simulink model "ec_single_vs_fixed"  (Simulink 10.0)
settings: Solver=FixedStepDiscrete  StartTime=0.0  StopTime=10  RelTol=1e-3
InitFcn:
  | ec_single_vs_fixed_data;
StartFcn:
  | tic;
StopFcn:
  | toc;
undefined symbols (not defined in the file): dfilt, ec_length, Fs, pic_frame_size, sm_length, spkr_to_mic_delay
libraries: dspsrcs4 x6, dspsigops x5, simulink x4, dspsnks4 x3, dspadpt3 x2, dsparch4 x1
settings Model: Creator=Kerry Schutz  LastModifiedBy=bhisma
settings DataIOCC: LimitDataPoints=on  SignalLoggingSaveFormat=ModelDataLogs
settings OptimizationCC: BlockReduction=off  DefaultParameterBehavior=Inlined  InlineInvariantSignals=on  ExpressionDepthLimit=2147483647  StateBitsets=on  DataBitsets=on  ZeroExternalMemoryAtStartup=off  ZeroInternalMemoryAtStartup=off  EfficientFloat2IntCast=on  LifeSpan=1  EfficientTunableParamExpr=on
settings DebuggingCC: AlgebraicLoopMsg=none  SaveWithParameterizedLinksMsg=none  SolverPrmCheckMsg=warning  ParameterPrecisionLossMsg=none  FcnCallInpInsideContextMsg=warning  StateNameClashWarn=warning
settings HardwareCC: ProdBitPerInt=16  ProdBitPerPointer=16  ProdBitPerSizeT=16  ProdBitPerPtrDiffT=16  ProdIntDivRoundTo=Zero  ProdEndianess=LittleEndian  ProdWordSize=16  ProdHWDeviceType=Microchip->dsPIC  TargetHWDeviceType=32-bit Generic
settings SFSimCC: SimUseLocalCustomCode=on  SimParseCustomCode=off  MATLABDynamicMemAlloc=off  CustomCodeUndefinedFunction=FilterOut
settings RTWCC: Description=Real-Time Workshop Embedded Coder (no auto configuration)  SystemTargetFile=ert.tlc  GenCodeOnly=on  TemplateMakefile=ert_default_tmf  RTWUseLocalCustomCode=on  CreateSILPILBlock=SIL
settings CodeAppCC: IgnoreCustomStorageClasses=off  CustomSymbolStrType=$N$R$M  InternalIdentifier=Classic  InlinedPrmAccess=Macros
settings ERTTargetCC: TargetFcnLib=ansi_tfl_tmw.mat  GenerateSampleERTMain=on  IncludeMdlTerminateFcn=off  SupportAbsoluteTime=off  PurelyIntegerCode=on  SupportNonFinite=off  SupportComplex=off  InlinedParameterPlacement=NonHierarchical  ERTCustomFileTemplate=example_file_process.tlc  ConvertIfToSwitch=off  SuppressUnreachableDefaultCases=off

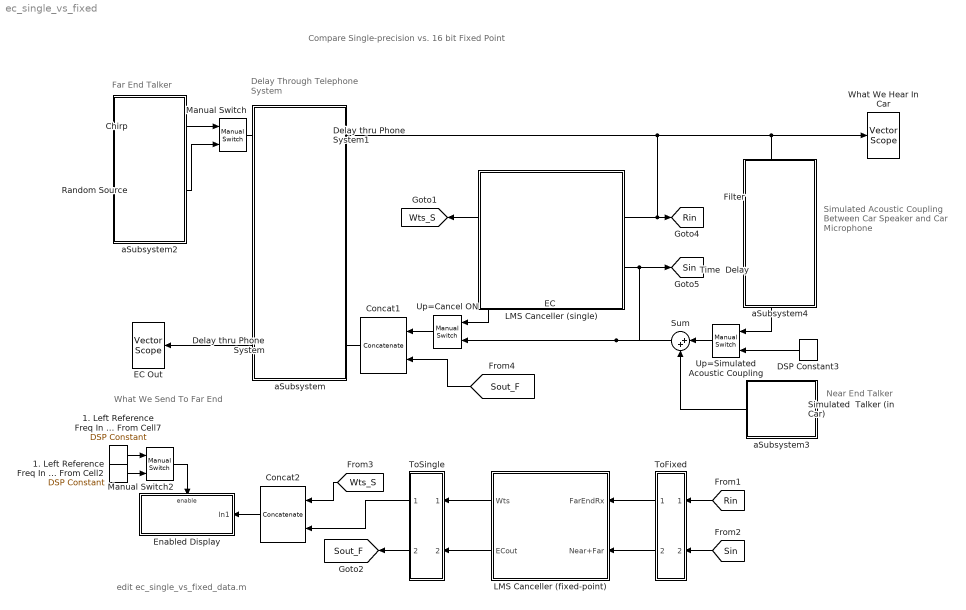
== system ec_single_vs_fixed ==
  note: Compare Single-precision vs. 16 bit Fixed Point
  note: Delay Through
      | Telephone System
  note: Simulated Acoustic
      | Coupling
      | Between Car Speaker
      | and
      | Car Microphone
  note: Far End Talker
  note: Near
      | End
      | Talker
  note: What We Send To
      | Far End
  note: edit ec_single_vs_fixed_data.m
  1. Left Reference Freq In Hz From Cell2 : dspsrcs4/DSP Constant  SystemSampleTime=-1  Value=0  SampleMode=Discrete  discreteOutput=Sample-based  continuousOutput=Sample-based  sampTime=pic_frame_size/Fs  framePeriod=pic_frame_size/Fs  dataType=int16  isSigned=on  wordLen=16  udDataType=sfix(16)  fracBitsMode=Best precision  numFracBits=15  InterpretAs1D=-inf  Ts=-inf  FramebasedOutput=-inf
      settings: SourceProductName=DSP System Toolbox  SourceProductBaseCode=DS  additionalParams=on
  1. Left Reference Freq In Hz From Cell7 : dspsrcs4/DSP Constant  SystemSampleTime=-1  Value=1  SampleMode=Discrete  discreteOutput=Sample-based  continuousOutput=Sample-based  sampTime=pic_frame_size/Fs  framePeriod=pic_frame_size/Fs  dataType=int16  isSigned=on  wordLen=16  udDataType=sfix(16)  fracBitsMode=Best precision  numFracBits=15  InterpretAs1D=-inf  Ts=-inf  FramebasedOutput=-inf
      settings: SourceProductName=DSP System Toolbox  SourceProductBaseCode=DS  additionalParams=on
  Chirp : dspsrcs4/Chirp  sweep=Linear  mode=Unidirectional  f0=100  f1=4000  t1=pic_frame_size/Fs  Tsweep=pic_frame_size/Fs  phase=0  Ts=1/Fs  spf=pic_frame_size  datatype=Single
      settings: SourceProductName=DSP System Toolbox
  Concat1 : Concatenate  Mode=Multidimensional array  ConcatenateDimension=2
  Concat2 : Concatenate  Mode=Multidimensional array  ConcatenateDimension=2
  DSP Constant3 : dspsrcs4/DSP Constant  SystemSampleTime=-1  Value=0  SampleMode=Discrete  discreteOutput=Sample-based  continuousOutput=Sample-based  sampTime=pic_frame_size/Fs  framePeriod=pic_frame_size/Fs  dataType=single  isSigned=on  wordLen=16  udDataType=sfix(16)  fracBitsMode=Best precision  numFracBits=15  InterpretAs1D=off  Ts=pic_frame_size/Fs  FramebasedOutput=off
      settings: SourceProductName=DSP System Toolbox  SourceProductBaseCode=DS
  Delay thru Phone System : dspsigops/Delay  dly_unit=Samples  delay=100  ic_detail=off  dif_ic_for_ch=off  dif_ic_for_dly=off  ic=0  reset_popup=None
      settings: SourceProductName=DSP System Toolbox  SourceProductBaseCode=DS
  Delay thru Phone System1 : dspsigops/Delay  dly_unit=Samples  delay=100  ic_detail=off  dif_ic_for_ch=off  dif_ic_for_dly=off  ic=0  reset_popup=None
      settings: SourceProductName=DSP System Toolbox  SourceProductBaseCode=DS
  EC : Subsystem
  EC Out : dspsnks4/Vector Scope  ScopeProperties=on  Domain=Time  HorizSpan=4  DisplayProperties=off  AxisGrid=on  Memory=off  FrameNumber=on  AxisLegend=on  AxisZoom=off  OpenScopeAtSimStart=on  OpenScopeImmediately=off  FigPos=[285 420 306 206]  AxisProperties=off  XUnits=Hertz  XRange=[0...Fs/2]  InheritXIncr=on  XIncr=1  XLabel=Time  XLimit=Auto  XMin=0  XMax=1  XStart=0  YUnits=dB  YLabel=Amplitude  LineProperties=off  LineColors=[1 0 0]|[0 1 0]
      settings: SourceProductName=DSP System Toolbox  SourceProductBaseCode=DS  YMin=-0.526783668994904  YMax=0.550434925854206
  Enabled Display : Subsystem  TreatAsAtomicUnit=on
  Filter : dsparch4/Digital Filter  Tag=BlockMethodSubSystem  TypePopup=FIR (all zeros)  IIRFiltStruct=Direct form II transposed  AllPoleFiltStruct=Direct form  FIRFiltStruct=Direct form  CoeffSource=Specify via dialog  NumCoeffs=spkr_to_mic_filter  DenCoeffs=[1 0.1]  BiQuadCoeffs=[1 0.3 0.4 1 0.1 0.2]  LatticeCoeffs=[0.2 0.4]  denIgnore=on  FiltPerSampPopup=One filter per frame  IC=0  ICnum=0  ICden=0  roundingMode=Floor  overflowMode=off  ScaleValues=1  scaleValueFracLength=14  stageInFracLength=15  stageOutFracLength=15  FilterSource=Specify via dialog  dfiltObjectName=dfilt.dffir([1 2 1])
      settings: SourceProductName=DSP System Toolbox  SourceProductBaseCode=DS
  LMS Canceller (fixed-point) : Subsystem  DataTypeOverride=Double  MinMaxOverflowLogging=MinMaxAndOverflow
  LMS Canceller (single) : Subsystem
      mask Display: disp('')
  Manual Switch : simulink/Signal Routing/Manual Switch  SystemSampleTime=-1  sw=0  action=0  varsize=off
      settings: SourceProductName=Simulink  SourceProductBaseCode=SL
  Manual Switch2 : simulink/Signal Routing/Manual Switch  SystemSampleTime=-1  sw=1  action=0  varsize=off
      settings: SourceProductName=Simulink  SourceProductBaseCode=SL
  Random Source : dspsrcs4/Random Source  SrcType=Gaussian  NormMethod=Ziggurat  CltLength=12  MinVal=0  MaxVal=1  MeanVal=0  VarVal=.2  RepMode=Repeatable  rawSeed=1  IsInherit=off  SampMode=Discrete  SampTime=1/Fs  SampFrame=pic_frame_size  DataType=Single  OutComplex=Real
  Simulated  Talker (in Car) : dspsrcs4/Sine Wave  Amplitude=0.2  Frequency=102  Phase=0  SampleMode=Discrete  OutComplex=Real  CompMethod=Trigonometric fcn  TableSize=Speed  SampleTime=1/Fs  SamplesPerFrame=pic_frame_size  dataType=single  wordLen=16  udDataType=sfix(16)  fracBitsMode=Best precision  numFracBits=15  ResetState=Restart at time zero
  Sum : Sum  Inputs=|++
  Time  Delay : dspsigops/Delay  dly_unit=Samples  delay=spkr_to_mic_delay  ic_detail=off  dif_ic_for_ch=off  dif_ic_for_dly=off  ic=0  reset_popup=None
      settings: SourceProductName=DSP System Toolbox  SourceProductBaseCode=DS
  ToFixed : Subsystem
  ToSingle : Subsystem
  Up=Cancel ON : simulink/Signal Routing/Manual Switch  SystemSampleTime=-1  sw=1  action=0  varsize=off
      settings: SourceProductName=Simulink  SourceProductBaseCode=SL
  Up=Simulated Acoustic Coupling : simulink/Signal Routing/Manual Switch  SystemSampleTime=-1  sw=1  action=0  varsize=off
      settings: SourceProductName=Simulink  SourceProductBaseCode=SL
  What We Hear In Car : dspsnks4/Vector Scope  ScopeProperties=on  Domain=Time  HorizSpan=1  DisplayProperties=off  AxisGrid=on  Memory=off  FrameNumber=on  AxisLegend=off  AxisZoom=off  OpenScopeAtSimStart=off  OpenScopeImmediately=off  FigPos=[77 319 306 206]  AxisProperties=off  XUnits=Hertz  XRange=[0...Fs/2]  InheritXIncr=on  XIncr=1  XLabel=Time  XLimit=Auto  XMin=0  XMax=1  XStart=0  YUnits=dB  YLabel=Amplitude  LineProperties=off
      settings: SourceProductName=DSP System Toolbox  SourceProductBaseCode=DS  YMin=-0.526783668994904  YMax=0.550434925854206
  aSubsystem : Subsystem
      mask Display: disp('')
  aSubsystem2 : Subsystem
      mask Display: disp('')
  aSubsystem3 : Subsystem
      mask Display: disp('')
  aSubsystem4 : Subsystem
      mask Display: disp('')
  tag scope: Rin=global, Sin=global, Sout_F=global, Wts_S=global
  wires:
  Chirp/1 -> Manual Switch/1
  Random Source/1 -> Manual Switch/2
  Manual Switch/1 -> Delay thru Phone System1/1
  Delay thru Phone System1/1 -> EC/1(FarEndRx), [Rin], What We Hear In Car/1, Filter/1
  Simulated  Talker (in Car)/1 -> Sum/2
  Up=Simulated Acoustic Coupling/1 -> Sum/1
  DSP Constant3/1 -> Up=Simulated Acoustic Coupling/2
  Sum/1 -> Up=Cancel ON/2, EC/2(Near+Far), [Sin]
  Time  Delay/1 -> Up=Simulated Acoustic Coupling/1
  EC/2(ECout) -> Up=Cancel ON/1
  Filter/1 -> Time  Delay/1
  ToFixed/1(Rin) -> LMS Canceller (fixed-point)/1(FarEndRx)
  ToFixed/2(Sin) -> LMS Canceller (fixed-point)/2(Near+Far)
  LMS Canceller (fixed-point)/1(Wts) -> ToSingle/1(In1)
  LMS Canceller (fixed-point)/2(ECout) -> ToSingle/2(In2)
  [Rin] -> ToFixed/1(In1)
  [Sin] -> ToFixed/2(" In2")
  Concat2/1 -> Enabled Display/1(In1)
  ToSingle/1(Wts) -> Concat2/2
  EC/1(Wts) -> [Wts_S]
  [Wts_S] -> Concat2/1
  ToSingle/2(Sout) -> [Sout_F]
  Up=Cancel ON/1 -> Concat1/1
  Concat1/1 -> Delay thru Phone System/1
  Delay thru Phone System/1 -> EC Out/1
  [Sout_F] -> Concat1/2
  1. Left Reference Freq In Hz From Cell7/1 -> Manual Switch2/1
  Manual Switch2/1 -> Enabled Display/Enable
  1. Left Reference Freq In Hz From Cell2/1 -> Manual Switch2/2

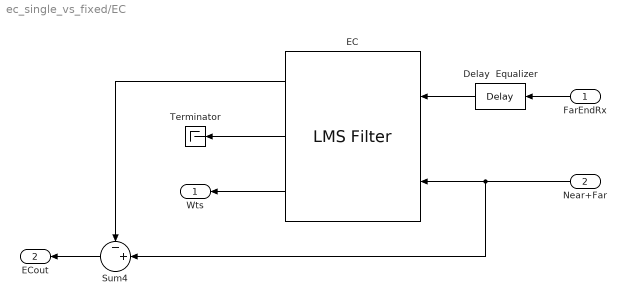
== system ec_single_vs_fixed/EC ==
  FarEndRx : Inport
  Near+Far : Inport  Port=2
  Delay  Equalizer : dspsigops/Delay  dly_unit=Samples  delay=spkr_to_mic_delay +sm_length/2 - 32/2  ic_detail=off  dif_ic_for_ch=off  dif_ic_for_dly=off  ic=0  reset_popup=None
      settings: SourceProductName=DSP System Toolbox  SourceProductBaseCode=DS
  EC : dspadpt3/LMS Filter  Algo=LMS  L=ec_length  stepflag=Dialog  mu=mu  leakage=1  ic=0  Adapt=off  resetflag=None  weights=on  secondCoeffMode=User-defined  secondCoeffWordLength=2  secondCoeffFracLength=14  accum2Mode=User-defined  accum2FracLength=30  prodOutput2Mode=User-defined  prodOutput2FracLength=15  prodOutput3Mode=User-defined  prodOutput3FracLength=15  prodOutput4Mode=User-defined  prodOutput4FracLength=15  quotientMode=User-defined  quotientFracLength=20  roundingMode=Nearest  overflowMode=off  addnparflag=off
      settings: SourceProductName=DSP System Toolbox  SourceProductBaseCode=DS
  Sum4 : Sum  Inputs=-+|  SaturateOnIntegerOverflow=on  InputSameDT=on  OutDataTypeStr=Inherit: Same as first input
  Terminator : Terminator
  Wts : Outport
  ECout : Outport  Port=2
  wires:
  Delay  Equalizer/1 -> EC/1
  FarEndRx/1 -> Delay  Equalizer/1
  Near+Far/1 -> EC/2, Sum4/2
  EC/1 -> Sum4/1
  EC/2 -> Terminator/1
  EC/3 -> Wts/1
  Sum4/1 -> ECout/1

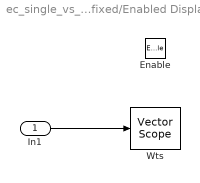
== system ec_single_vs_fixed/Enabled Display ==
  In1 : Inport
  Enable : EnablePort
  Wts : dspsnks4/Vector Scope  ScopeProperties=on  Domain=Time  HorizSpan=1  DisplayProperties=off  AxisGrid=on  Memory=off  FrameNumber=on  AxisLegend=on  AxisZoom=off  OpenScopeAtSimStart=on  OpenScopeImmediately=off  FigPos=[599 420 306 206]  AxisProperties=off  XUnits=Hertz  XRange=[0...Fs/2]  InheritXIncr=on  XIncr=1  XLabel=Time  XLimit=Auto  XMin=0  XMax=1  XStart=0  YUnits=dB  YLabel=Amplitude  LineProperties=off  LineColors=[1 0 0]|[0 1 0]
      settings: SourceProductName=DSP System Toolbox  SourceProductBaseCode=DS  YMin=-0.526783668994904  YMax=0.550434925854206
  wires:
  In1/1 -> Wts/1

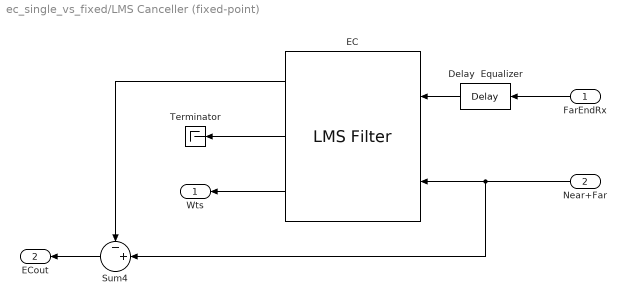
== system ec_single_vs_fixed/LMS Canceller (fixed-point) ==
  FarEndRx : Inport
  Near+Far : Inport  Port=2
  Delay  Equalizer : dspsigops/Delay  dly_unit=Samples  delay=spkr_to_mic_delay +sm_length/2 - ec_length/2  ic_detail=off  dif_ic_for_ch=off  dif_ic_for_dly=off  ic=0  reset_popup=None
      settings: SourceProductName=DSP System Toolbox  SourceProductBaseCode=DS
  EC : dspadpt3/LMS Filter  Algo=LMS  L=ec_length  stepflag=Dialog  mu=mu  leakage=1  ic=0  Adapt=off  resetflag=None  weights=on  firstCoeffMode=Binary point scaling  firstCoeffWordLength=16  firstCoeffFracLength=15  secondCoeffMode=User-defined  secondCoeffWordLength=2  secondCoeffFracLength=15  accumMode=Binary point scaling  accumWordLength=32  accumFracLength=20  accum2Mode=User-defined  accum2FracLength=20  prodOutputMode=Binary point scaling  prodOutputWordLength=16  prodOutputFracLength=20  prodOutput2Mode=User-defined  prodOutput2FracLength=15  prodOutput3Mode=User-defined  prodOutput3FracLength=15  prodOutput4Mode=User-defined  prodOutput4FracLength=15  quotientMode=User-defined  quotientFracLength=20  memoryMode=Binary point scaling  memoryWordLength=16  memoryFracLength=15  roundingMode=Nearest  overflowMode=off  addnparflag=off
      settings: SourceProductName=DSP System Toolbox  SourceProductBaseCode=DS
  Sum4 : Sum  Inputs=-+|  SaturateOnIntegerOverflow=on  InputSameDT=on  OutDataTypeStr=Inherit: Same as first input
  Terminator : Terminator
  Wts : Outport
  ECout : Outport  Port=2
  wires:
  Sum4/1 -> ECout/1
  EC/3 -> Wts/1
  EC/2 -> Terminator/1
  EC/1 -> Sum4/1
  Near+Far/1 -> Sum4/2, EC/2
  FarEndRx/1 -> Delay  Equalizer/1
  Delay  Equalizer/1 -> EC/1

== system ec_single_vs_fixed/LMS Canceller (single) ==

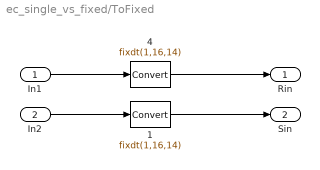
== system ec_single_vs_fixed/ToFixed ==
  In1 : Inport
  " In2" : Inport  Port=2
  " 1" : DataTypeConversion  OutDataTypeStr=fixdt(1,16,14)
  " 4" : DataTypeConversion  OutDataTypeStr=fixdt(1,16,14)
  Rin : Outport
  Sin : Outport  Port=2
  wires:
  " 1"/1 -> Sin/1
  " In2"/1 -> " 1"/1
  " 4"/1 -> Rin/1
  In1/1 -> " 4"/1

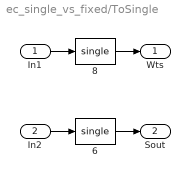
== system ec_single_vs_fixed/ToSingle ==
  In1 : Inport
  In2 : Inport  Port=2
  " 6" : DataTypeConversion  OutDataTypeStr=single
  " 8" : DataTypeConversion  OutDataTypeStr=single
  Wts : Outport
  Sout : Outport  Port=2
  wires:
  " 6"/1 -> Sout/1
  In2/1 -> " 6"/1
  " 8"/1 -> Wts/1
  In1/1 -> " 8"/1

== system ec_single_vs_fixed/aSubsystem ==

== system ec_single_vs_fixed/aSubsystem2 ==

== system ec_single_vs_fixed/aSubsystem3 ==

== system ec_single_vs_fixed/aSubsystem4 ==
